simulink model "IBC2019"  (R2019b)
settings: Solver=VariableStepAuto  StartTime=0.0  StopTime=0.01  RelTol=1e-3
libraries: simulink x7, spsSeriesRLCBranchLib x4, spsCurrentMeasurementLib x4, spsDiodeLib x3, spsMosfetLib x3, dspsigops x2, spsParallelRLCBranchLib x1, spsDCVoltageSourceLib x1, spsVoltageMeasurementLib x1, spspowerguiLib x1
settings Model: Creator=29721  LastModifiedBy=Dell
settings SolverCC: ZeroCrossAlgorithm=Adaptive
settings DebuggingCC: IgnoredZcDiagnostic=none

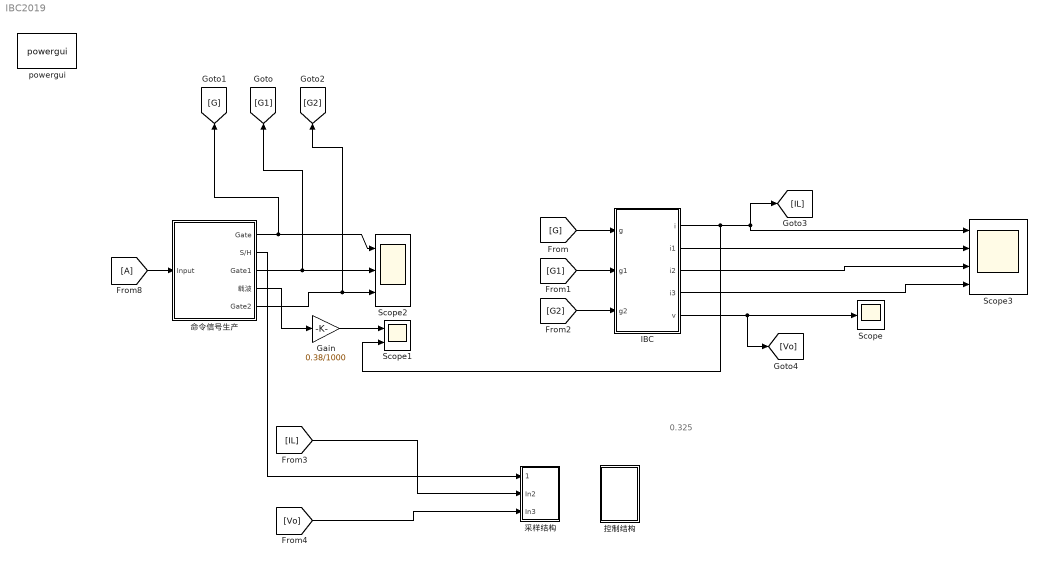
== system IBC2019 ==
  note: 0.325
  Gain : Gain  Gain=0.38/1000
  IBC : Subsystem  mask{Vin=15, C=9e-8, Load=60, L=2.332e-3}
  Scope : Scope
  Scope1 : Scope  NumInputPorts=2
  Scope2 : Scope  NumInputPorts=3
  Scope3 : Scope  NumInputPorts=4
  powergui : spspowerguiLib/powergui  Priority=1  SimulationMode=Discrete  SampleTime=2.5e-8  frequency=60  Iterations=50  frequencyindice=0  Pbase=100e6  ErrMax=1e-4  UnitsV=kV  UnitsW=MW  buscounter=0  FunctionMessages=off  echomessages=off  EnableUseOfTLC=off  CurrentSourceSwitches=on  DisableSnubberDevices=off  DisableRonSwitches=off  DisableVfSwitches=off  DisplayEquations=off  AutomaticDiscreteSolvers=off  SolverType=Tustin  Interpol=off  ExternalGateDelay=off  methode=off  Ts=100  x0status=blocks  SPID=off  SwTol=0  HookPort=off  NonlinearTolerance=1e-4  nMaxIteration=100  ContinueOnMaxIteration=off  RestoreLinks=warning  ResistiveCurrentMeasurement=off  Frange=[0:2:500]  Ylog=off  Xlog=on  ShowGrid=off  save=off  variable=ZData  structure=ScopeData  ZoomFFT=off  StartTime=0.033333  cycles=1  DisplayStyle=1  fundamental=300000  FreqAxis=on  MaxFrequency=300000  frequencyindicesteady=1  RmsSteady=1  display=off
  命令信号生产 : Subsystem  mask{Fs=100e3}
      mask prompts: Fs "swicthing frequency"
  控制结构 : Subsystem
  采样结构 : Subsystem
  wires:
  命令信号生产/1(Gate) -> Scope2/1, [G]
  命令信号生产/3(Gate1) -> Scope2/2, [G1]
  命令信号生产/5(Gate2) -> Scope2/3, [G2]
  IBC/1(i) -> Scope1/2, Scope3/1, [IL]
  IBC/2(i1) -> Scope3/2
  IBC/3(i2) -> Scope3/3
  IBC/4(i3) -> Scope3/4
  IBC/5(v) -> [Vo], Scope/1
  [A] -> 命令信号生产/1(Input)
  命令信号生产/4(载波) -> Gain/1
  [G] -> IBC/1(g)
  [G1] -> IBC/2(g1)
  [G2] -> IBC/3(g2)
  Gain/1 -> Scope1/1
  命令信号生产/2(S/H) -> 采样结构/1(Trigger)
  [IL] -> 采样结构/2(In2)
  [Vo] -> 采样结构/3(In3)

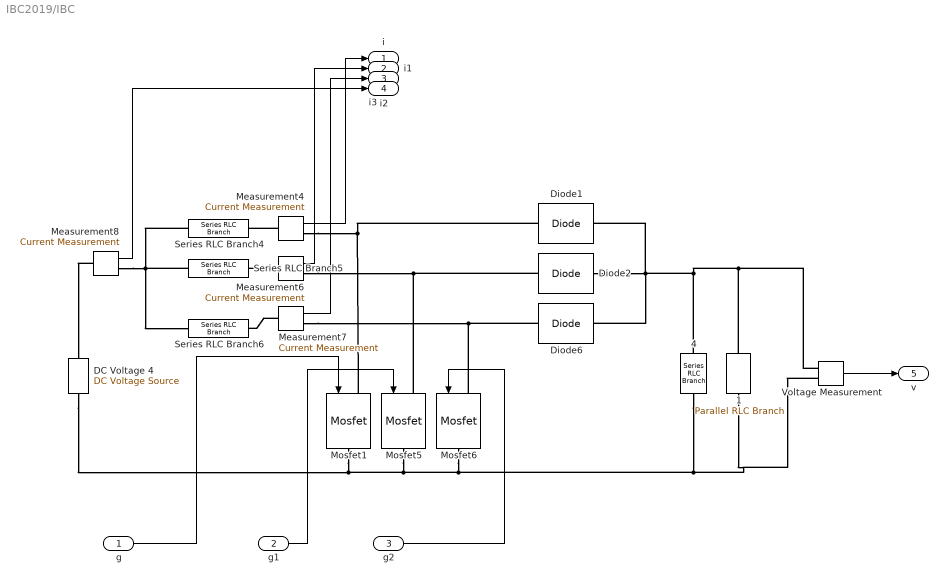
== system IBC2019/IBC ==
  g : Inport
  g1 : Inport  Port=2
  g2 : Inport  Port=3
  "    4" : spsSeriesRLCBranchLib/Series RLC Branch  LConnTagsString=__new0  RConnTagsString=__new0  BranchType=C  Resistance=0  Inductance=69e-3  SetiL0=off  InitialCurrent=0  Capacitance=C  Setx0=off  InitialVoltage=0  Measurements=None
  "  1" : spsParallelRLCBranchLib/Parallel RLC Branch  LConnTagsString=a  RConnTagsString=__new0  BranchType=R  Resistance=Load  Inductance=1e-3  SetiL0=off  InitialCurrent=0  Capacitance=1e-6  Setx0=off  InitialVoltage=0  Measurements=None
   Measurement{4,6..8} (4 alike) : spsCurrentMeasurementLib/Current Measurement  PhasorSimulation=off  OutputType=Complex  PSBequivalent=0
  DC Voltage 4 : spsDCVoltageSourceLib/DC Voltage Source  Amplitude=Vin  Measurements=Voltage
  Diode1 : spsDiodeLib/Diode  Ron=0.001  Lon=0  Vf=0.8  IC=0  UseSnubber=off  Rs=inf  Cs=250e-9  Measurements=off
  Diode2 : spsDiodeLib/Diode  Ron=0.001  Lon=0  Vf=0.8  IC=0  UseSnubber=off  Rs=inf  Cs=250e-9  Measurements=off
  Diode6 : spsDiodeLib/Diode  Ron=0.001  Lon=0  Vf=0.8  IC=0  UseSnubber=off  Rs=inf  Cs=250e-9  Measurements=off
  Mosfet1 : spsMosfetLib/Mosfet  Ron=0.1  Lon=0  Rd=0.01  Vfd=0  IC=0  Rs=1e5  Cs=inf  Measurements=off
  Mosfet5 : spsMosfetLib/Mosfet  Ron=0.1  Lon=0  Rd=0.01  Vfd=0  IC=0  Rs=1e5  Cs=inf  Measurements=off
  Mosfet6 : spsMosfetLib/Mosfet  Ron=0.1  Lon=0  Rd=0.01  Vfd=0  IC=0  Rs=1e5  Cs=inf  Measurements=off
  Series RLC Branch4 : spsSeriesRLCBranchLib/Series RLC Branch  LConnTagsString=__new0  RConnTagsString=__new0  BranchType=L  Resistance=0  Inductance=L  SetiL0=off  InitialCurrent=0  Capacitance=1e-6  Setx0=off  InitialVoltage=0  Measurements=None
  Series RLC Branch5 : spsSeriesRLCBranchLib/Series RLC Branch  LConnTagsString=__new0  RConnTagsString=__new0  BranchType=L  Resistance=0  Inductance=L  SetiL0=off  InitialCurrent=0  Capacitance=1e-6  Setx0=off  InitialVoltage=0  Measurements=None
  Series RLC Branch6 : spsSeriesRLCBranchLib/Series RLC Branch  LConnTagsString=__new0  RConnTagsString=__new0  BranchType=L  Resistance=0  Inductance=L  SetiL0=off  InitialCurrent=0  Capacitance=1e-6  Setx0=off  InitialVoltage=0  Measurements=None
  Voltage Measurement : spsVoltageMeasurementLib/Voltage Measurement  PhasorSimulation=off  OutputType=Complex  PSBequivalent=0
  i : Outport
  i1 : Outport  Port=2
  i2 : Outport  Port=3
  i3 : Outport  Port=4
  v : Outport  Port=5
  wires:
  g1/1 -> Mosfet5/1
  g2/1 -> Mosfet6/1
  " Measurement4"/1 -> i/1
  " Measurement8"/1 -> i3/1
  " Measurement6"/1 -> i1/1
  Voltage Measurement/1 -> v/1
  g/1 -> Mosfet1/1
  " Measurement7"/1 -> i2/1
  connections:
  " Measurement7"/RConn1 -- Diode6/LConn1 -- Mosfet6/LConn1
  " Measurement6"/RConn1 -- Diode2/LConn1 -- Mosfet5/LConn1
  " Measurement8"/LConn1 -- DC Voltage 4/RConn1
  Voltage Measurement/LConn2 -- "  1"/RConn1 -- "    4"/RConn1 -- Mosfet6/RConn1 -- Mosfet5/RConn1 -- Mosfet1/RConn1 -- DC Voltage 4/LConn1
  Series RLC Branch4/LConn1 -- Series RLC Branch5/LConn1 -- Series RLC Branch6/LConn1 -- " Measurement8"/RConn1
  " Measurement4"/LConn1 -- Series RLC Branch4/RConn1
  " Measurement6"/LConn1 -- Series RLC Branch5/RConn1
  " Measurement7"/LConn1 -- Series RLC Branch6/RConn1
  Diode1/LConn1 -- Mosfet1/LConn1 -- " Measurement4"/RConn1
  Voltage Measurement/LConn1 -- "    4"/LConn1 -- Diode6/RConn1 -- Diode2/RConn1 -- Diode1/RConn1 -- "  1"/LConn1

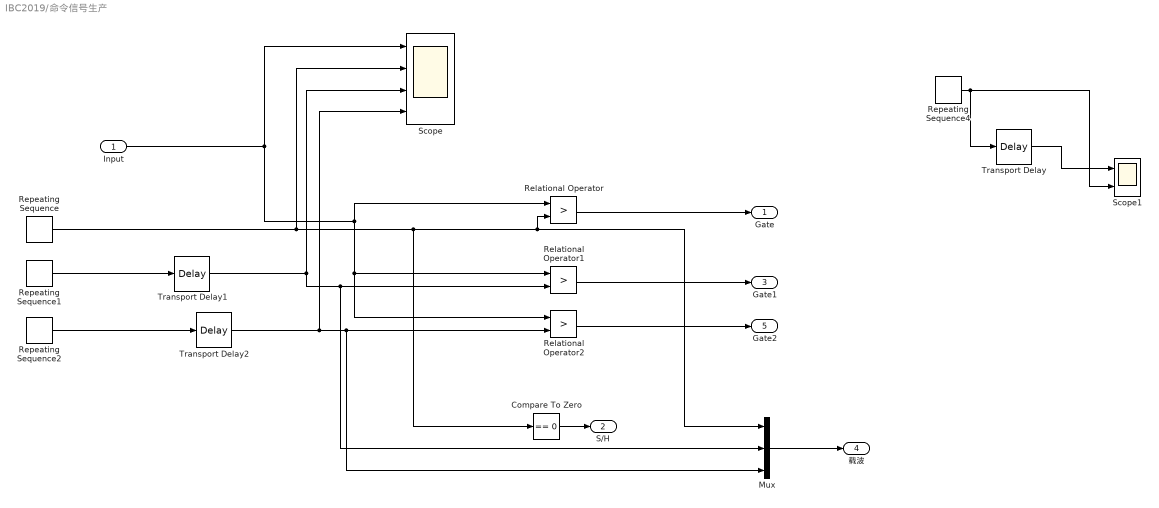
== system IBC2019/命令信号生产 ==
  Input : Inport
  Compare To Zero : simulink/Logic and Bit Operations/Compare To Zero  relop===  OutDataTypeStr=boolean
  Mux : Mux  Inputs=3
  Relational Operator : RelationalOperator  Operator=>  OutDataTypeStr=boolean  RndMeth=Simplest
  Relational Operator1 : RelationalOperator  Operator=>  OutDataTypeStr=boolean  RndMeth=Simplest
  Relational Operator2 : RelationalOperator  Operator=>  OutDataTypeStr=boolean  RndMeth=Simplest
  Repeating Sequence : simulink/Sources/Repeating Sequence  rep_seq_t=[0 1./Fs./2 1./Fs]  rep_seq_y=[0 1000 0]
  Repeating Sequence1 : simulink/Sources/Repeating Sequence  rep_seq_t=[1./Fs./3 5./Fs./6 4./Fs./3]  rep_seq_y=[0 1000 0]
  Repeating Sequence2 : simulink/Sources/Repeating Sequence  rep_seq_t=[2./Fs./3 7./Fs./6 5./Fs./3]  rep_seq_y=[0 1000 0]
  Repeating Sequence4 : simulink/Sources/Repeating Sequence  rep_seq_t=[0 1./100e3./2 1./100e3]  rep_seq_y=[0 1000 0]
  Scope : Scope  NumInputPorts=4
  Scope1 : Scope  NumInputPorts=2
  Transport Delay : TransportDelay  DelayTime=1./100e3./3
  Transport Delay1 : TransportDelay  DelayTime=1./100e3./3
  Transport Delay2 : TransportDelay  DelayTime=2./100e3./3
  Gate : Outport
  S/H : Outport  Port=2
  Gate1 : Outport  Port=3
  载波 : Outport  Port=4
  Gate2 : Outport  Port=5
  wires:
  Input/1 -> Relational Operator1/1, Relational Operator2/1, Relational Operator/1, Scope/1
  Compare To Zero/1 -> S/H/1
  Relational Operator/1 -> Gate/1
  Repeating Sequence/1 -> Scope/2, Mux/1, Relational Operator/2, Compare To Zero/1
  Repeating Sequence1/1 -> Transport Delay1/1
  Relational Operator1/1 -> Gate1/1
  Repeating Sequence2/1 -> Transport Delay2/1
  Mux/1 -> 载波/1
  Relational Operator2/1 -> Gate2/1
  Repeating Sequence4/1 -> Transport Delay/1, Scope1/2
  Transport Delay/1 -> Scope1/1
  Transport Delay1/1 -> Mux/2, Relational Operator1/2, Scope/3
  Transport Delay2/1 -> Scope/4, Mux/3, Relational Operator2/2

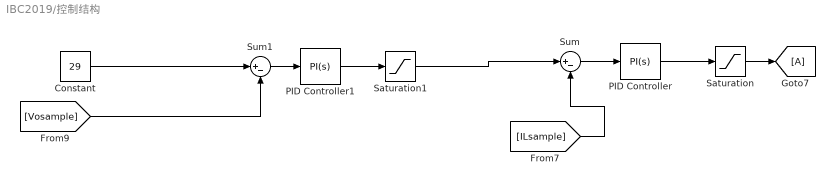
== system IBC2019/控制结构 ==
  Constant : Constant  Value=29
  PID Controller : simulink/Continuous/PID Controller  Controller=PI  Form=Parallel  TimeDomain=Continuous-time  SampleTime=-1  IntegratorMethod=Forward Euler  ControllerParametersSource=internal  P=1039.7331488904  I=55419501.5119954  D=0  UseFilter=on  N=100  TunerSelectOption=Transfer Function Based (PID Tuner App)  InitialConditionSource=internal  InitialConditionForIntegrator=0  InitialConditionForFilter=0  DifferentiatorICPrevScaledInput=0  ExternalReset=none  TrackingMode=off  Kt=1  LimitOutput=off  UpperSaturationLimit=inf  LowerSaturationLimit=-inf  LinearizeAsGain=on  AntiWindupMode=none  Kb=1  POutMin=[]  POutMax=[]  IOutMin=[]  IOutMax=[]  DOutMin=[]  DOutMax=[]  NOutMin=[]  NOutMax=[]  SumOutMin=[]  SumOutMax=[]  SaturationOutMin=[]  SaturationOutMax=[]  PParamMin=[]  PParamMax=[]  IParamMin=[]  IParamMax=[]  DParamMin=[]  DParamMax=[]  NParamMin=[]  NParamMax=[]  KbParamMin=[]  KbParamMax=[]  KtParamMin=[]  KtParamMax=[]  KbOutMin=[]  KbOutMax=[]  KtOutMin=[]  KtOutMax=[]  IntegratorOutMin=[]  IntegratorOutMax=[]  FilterOutMin=[]  FilterOutMax=[]  SumI1OutMin=[]  SumI1OutMax=[]  SumI2OutMin=[]  SumI2OutMax=[]  SumI3OutMin=[]  SumI3OutMax=[]  SumI4OutMin=[]  SumI4OutMax=[]  SumDOutMin=[]  SumDOutMax=[]  DifferentiatorOutMin=[]  DifferentiatorOutMax=[]  FilterDiffOutCoefMin=[]  FilterDiffOutCoefMax=[]  ReciprocalOutMin=[]  ReciprocalOutMax=[]  SumDenOutMin=[]  SumDenOutMax=[]  SumNumOutMin=[]  SumNumOutMax=[]  DivideOutMin=[]  DivideOutMax=[]  IntegratorContinuousStateAttributes=''  IntegratorStateMustResolveToSignalObject=off  IntegratorRTWStateStorageClass=Auto  FilterContinuousStateAttributes=''  FilterStateMustResolveToSignalObject=off  FilterRTWStateStorageClass=Auto  ParallelPVariant=InternalParameters  IdealPVariant=Disabled  IVariant=InternalParameters  DVariant=Disabled  IntegratorVariant=Continuous  SatVariant=Disabled  AWVariant=Passthrough  PCopyVariant=Disabled  TRVariant=Disabled  FdbkBlocksVariant=Forward  IdealPFdbkVariant=Disabled  SatFdbkVariant=Disabled  DerivativeFilterVariant=Disabled  NVariant=Disabled  NCopyVariant=Disabled_SignalSpec  FilterICVariant=Disabled  IntegratorICVariant=InternalICs  ExternalResetVariant=Disabled  TRSumVariant=Passthrough  SumFdbkVariant=Disabled  SumVariant=Sum_PI
  PID Controller1 : simulink/Continuous/PID Controller  Controller=PI  Form=Parallel  TimeDomain=Continuous-time  SampleTime=-1  IntegratorMethod=Forward Euler  ControllerParametersSource=internal  P=0.01  I=10  D=0  UseFilter=on  N=100  TunerSelectOption=Transfer Function Based (PID Tuner App)  InitialConditionSource=internal  InitialConditionForIntegrator=0  InitialConditionForFilter=0  DifferentiatorICPrevScaledInput=0  ExternalReset=none  TrackingMode=off  Kt=1  LimitOutput=off  UpperSaturationLimit=inf  LowerSaturationLimit=-inf  LinearizeAsGain=on  AntiWindupMode=none  Kb=1  POutMin=[]  POutMax=[]  IOutMin=[]  IOutMax=[]  DOutMin=[]  DOutMax=[]  NOutMin=[]  NOutMax=[]  SumOutMin=[]  SumOutMax=[]  SaturationOutMin=[]  SaturationOutMax=[]  PParamMin=[]  PParamMax=[]  IParamMin=[]  IParamMax=[]  DParamMin=[]  DParamMax=[]  NParamMin=[]  NParamMax=[]  KbParamMin=[]  KbParamMax=[]  KtParamMin=[]  KtParamMax=[]  KbOutMin=[]  KbOutMax=[]  KtOutMin=[]  KtOutMax=[]  IntegratorOutMin=[]  IntegratorOutMax=[]  FilterOutMin=[]  FilterOutMax=[]  SumI1OutMin=[]  SumI1OutMax=[]  SumI2OutMin=[]  SumI2OutMax=[]  SumI3OutMin=[]  SumI3OutMax=[]  SumI4OutMin=[]  SumI4OutMax=[]  SumDOutMin=[]  SumDOutMax=[]  DifferentiatorOutMin=[]  DifferentiatorOutMax=[]  FilterDiffOutCoefMin=[]  FilterDiffOutCoefMax=[]  ReciprocalOutMin=[]  ReciprocalOutMax=[]  SumDenOutMin=[]  SumDenOutMax=[]  SumNumOutMin=[]  SumNumOutMax=[]  DivideOutMin=[]  DivideOutMax=[]  IntegratorContinuousStateAttributes=''  IntegratorStateMustResolveToSignalObject=off  IntegratorRTWStateStorageClass=Auto  FilterContinuousStateAttributes=''  FilterStateMustResolveToSignalObject=off  FilterRTWStateStorageClass=Auto  ParallelPVariant=InternalParameters  IdealPVariant=Disabled  IVariant=InternalParameters  DVariant=Disabled  IntegratorVariant=Continuous  SatVariant=Disabled  AWVariant=Passthrough  PCopyVariant=Disabled  TRVariant=Disabled  FdbkBlocksVariant=Forward  IdealPFdbkVariant=Disabled  SatFdbkVariant=Disabled  DerivativeFilterVariant=Disabled  NVariant=Disabled  NCopyVariant=Disabled_SignalSpec  FilterICVariant=Disabled  IntegratorICVariant=InternalICs  ExternalResetVariant=Disabled  TRSumVariant=Passthrough  SumFdbkVariant=Disabled  SumVariant=Sum_PI
  Saturation : Saturate  UpperLimit=900  LowerLimit=100
  Saturation1 : Saturate  UpperLimit=0.4  LowerLimit=0.3
  Sum : Sum  Inputs=|+-
  Sum1 : Sum  Inputs=|+-
  wires:
  PID Controller1/1 -> Saturation1/1
  Saturation/1 -> [A]
  [ILsample] -> Sum/2
  Sum/1 -> PID Controller/1
  PID Controller/1 -> Saturation/1
  [Vosample] -> Sum1/2
  Saturation1/1 -> Sum/1
  Constant/1 -> Sum1/1
  Sum1/1 -> PID Controller1/1

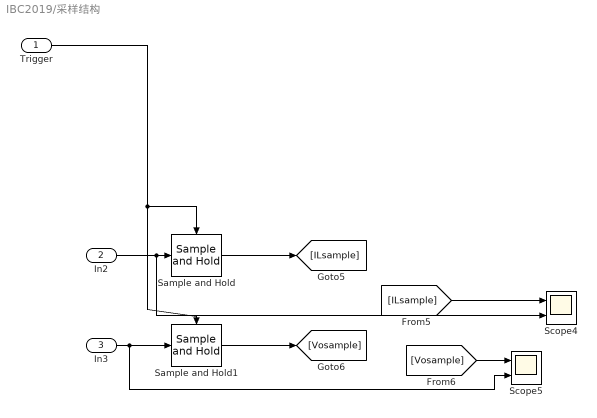
== system IBC2019/采样结构 ==
  Trigger : Inport
  In2 : Inport  Port=2
  In3 : Inport  Port=3
  Sample and Hold : dspsigops/Sample and Hold  trig=Rising edge  initCond=0  latchinput=off
  Sample and Hold1 : dspsigops/Sample and Hold  trig=Rising edge  initCond=0  latchinput=off
  Scope4 : Scope  NumInputPorts=2
  Scope5 : Scope  NumInputPorts=2
  wires:
  Sample and Hold1/1 -> [Vosample]
  Trigger/1 -> Sample and Hold1/Trigger, Sample and Hold/Trigger
  Sample and Hold/1 -> [ILsample]
  [Vosample] -> Scope5/1
  [ILsample] -> Scope4/1
  In3/1 -> Scope5/2, Sample and Hold1/1
  In2/1 -> Scope4/2, Sample and Hold/1
